simulink model "MCLV_Board_33Fj256MC710A_BLDC_wHall_async_2_10Khz"  (Simulink 7.5)
settings: Solver=FixedStepDiscrete  StartTime=0.0  StopTime=10.0  FixedStep=.001  RelTol=1e-3
undefined symbols (not defined in the file or in its folder): CN19max, D13, D14, D15, DiscIntNeverNeededParam, F13, Max, ms, Pin, PWM1max, PWMmax, Resol, us
libraries: MCHP_Blockset x17, simulink x8
CloseFcn:
  | rtwprivate ssgencode ModelCloseRequest MCLV_Board_33Fj256MC710A_BLDC_wHall_async_2_10Khz
settings Model: Creator=Lubin Kerhuel  LastModifiedBy=Lubin Kerhuel
settings OptimizationCC: InlineParams=on  InlineInvariantSignals=on  EnhancedBackFolding=on  OptimizeModelRefInitCode=on  LifeSpan=1
settings HardwareCC: ProdBitPerInt=16  ProdIntDivRoundTo=Zero  ProdEndianess=LittleEndian  ProdWordSize=16  ProdHWDeviceType=Generic->Custom
settings ModelReferenceCC: ModelReferenceNumInstancesAllowed=Single
settings RTWCC: SystemTargetFile=MCHP_dsPIC_stf.tlc  TemplateMakefile=MCHP_dsPIC.tmf  Description=Microchip Embedded Target PIC24 dsPIC30 dsPIC33 (real-time)  GenerateReport=on  ProcessScript=MCHP_dsPIC_stf_make_rtw_hook  IncludeHyperlinkInReport=on  GenerateTraceInfo=on  GenerateTraceReport=on  GenerateTraceReportSl=on  GenerateTraceReportSf=on  GenerateTraceReportEml=on
settings CodeAppCC: IgnoreCustomStorageClasses=off  MaxIdLength=255
settings STFCustomTargetCC: TargetLibSuffix=_lib.a  IncludeMdlTerminateFcn=off  CombineOutputUpdateFcns=on  SuppressErrorStatus=on  ERTCustomFileBanners=on  SupportContinuousTime=off  SystemTargetFile=MCHP_dsPIC_stf.tlc
settings ERTTargetCC: TargetLibSuffix=_lib.a  MultiwordLength=2048  ParMdlRefBuildCompliant=off  CompOptLevelCompliant=off  IncludeMdlTerminateFcn=off  SuppressErrorStatus=on  ERTFirstTimeCompliant=off  SupportNonInlinedSFcns=on  ModelStepFunctionPrototypeControlCompliant=off  CPPClassGenCompliant=off  InlinedParameterPlacement=NonHierarchical  ERTSrcFileBannerTemplate=MCHP_dsPIC_code_template.cgt  ERTHdrFileBannerTemplate=MCHP_dsPIC_code_template.cgt  ERTDataSrcFileTemplate=MCHP_dsPIC_code_template.cgt  ERTDataHdrFileTemplate=MCHP_dsPIC_code_template.cgt  ERTCustomFileTemplate=MCHP_main.tlc  ConvertIfToSwitch=off
settings CustomProperty: DataType=string  Value=33FJ256MC710A
settings EnumStrPairs: String=elf

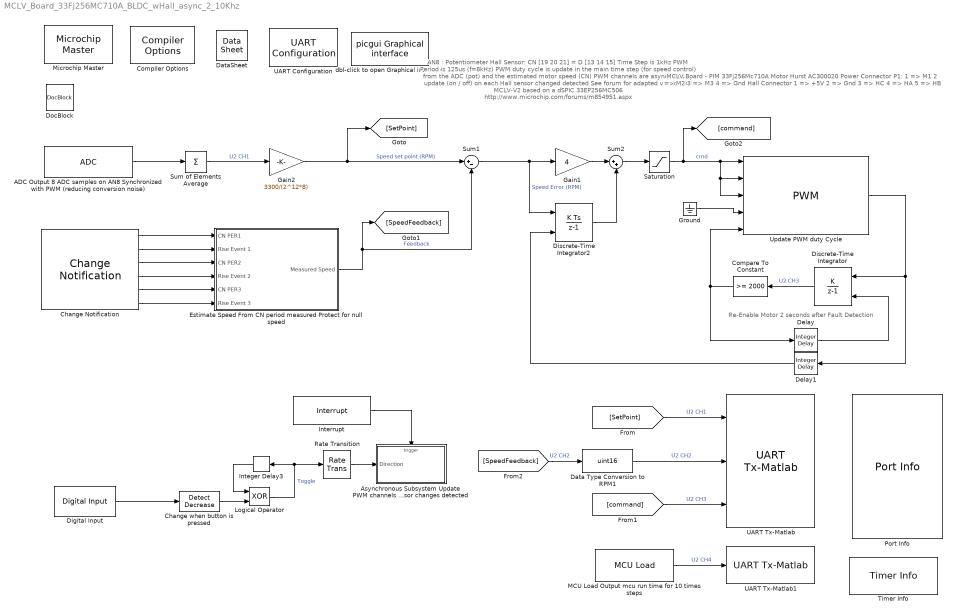
== system MCLV_Board_33Fj256MC710A_BLDC_wHall_async_2_10Khz ==
  note: Re-Enable Motor 2 seconds after Fault Detection
  note: AN8 : Potentiometer
      | Hall Sensor: CN [19 20 21] = D [13 14 15]
      |
      | Time Step is 1kHz
      | PWM Period is 125us (f=8kHz)
      | PWM duty cycle is update in the main time step (for speed control)
      | from the ADC (pot) and the estimated motor speed (CN)
      | PWM channels are asynchrousnly update (on / off) on each Hall sensor changed detected
      |
      | See forum for adapted version for MCLV-V2 based on a dSPIC 33EP256MC506
      | http://www.microchip.com/forums/m854951.aspx
  note: MCLV Board -  PIM 33Fj256Mc710A
      | Motor Hurst AC300020
      | Power Connector P1:
      | 1 => M1
      | 2 => M2
      | 3 => M3
      | 4 => Gnd
      | Hall Connector
      | 1 => +5V
      | 2 => Gnd
      | 3 => HC
      | 4 => HA
      | 5 => HB
  ADC Output 8 ADC samples on AN8 Synchronized with PWM (reducing conversion noise) : MCHP_Blockset/Analog IO/ADC  ADC_REF=1  Mode=12 bits  FORM=0000 dddd dddd dddd ==> Unsigned integer  nSAMPLECHANNELS=CH0 only  nSAMPLECHANNELS_12bits=CH0 only  SIMULTANEOUS=in Sequence  ADxCSS=8  MUXA_CH0N=off  MUXA_CH123=Dynamic Options  MUXA_CH123_TXT=AN0 : AN1 : AN2  MUXB_CH0=AN1  MUXB_CH0N=on  MUXB_CH123=Dynamic Options  MUXB_CH123_TXT=AN0 : AN1 : AN2  SequenceRepeat=8  SequenceTiming=are done as fast as possible ; triggered by user define source  SSRC_SSRCG=Dynamic Options  SSRC_SSRCG_TXT=6  Update_BlockOutput=After all trig and conversion sequence  Trig_TimeStep=with each update of the ADC block output  ADC_DMA_CHANNEL=use DMA Channel 1  SampleTime=0.001  Info=Total Time for Sample & Conversion : 7.56e-005s including 0s (x 8) sample time.  MCHP_PORT={Analog Input 8}{AN8}15:2:B8;  MCHP_MASTERLINK=MCLV_Board_33Fj256MC710A_BLDC_wHall_async_2_10Khz/Microchip Master  ADC_TIMING=[7.5599999999999994e-005]
  Asynchronous Subsystem Update PWM channels to On / Off based on Hall sensor changes detected : Subsystem
  Change Notification : MCHP_Blockset/Pulse Input//Output/Change Notification  IntPriority=6  Channel="[19    20    21]"  Channel_EP="[  D13  D14  D15 ]"  Channel_OLD="[19  20  21]"  Channel_UP_Down_Periode="[4     4     4]"  MaxChannel="[0.25   0.25   0.25]"  SafeMarge="[200   200   200]"  MaxChannelValue="2.^[ 15.253  15.253  15.253]  =>  [39062  39062  39062]"  CNxmax="[39062  39062  39062]"  Timer="[2  2  2]"  ChangeDetected="[1     1     1]"  OutputPortValue="[0     0     0]"  SampleTime=.001  Status=OK  MCHP_PORT={Change Notification 19}{CN19}9:0:D13;{Change Notification 20}{CN20}9:0:D14;{Change Notification 21}{CN21}9:0:D15;  MCHP_TIMER_REQUEST={Change Notification 19}{CN19}7:1:1:0:[]:30000000;{Change Notification 20}{CN20}7:1:1:0:[]:30000000;{Change Notification 21}{CN21}7:1:1:0:[]:30000000;  MCHP_TIMER_RESULT=[2 117186.50000000007 ;2 117186.50000000007 ;2 117186.50000000007 ]  MCHP_USER_INTERRUPTS={CNIE}{CN}{Change Notification}{6};  MCHP_MASTERLINK=MCLV_Board_33Fj256MC710A_BLDC_wHall_async_2_10Khz/Microchip Master
  Change when button is pressed : simulink/Logic and Bit Operations/Detect Decrease  SystemSampleTime=-1  vinit=0.0
  Compare To Constant : simulink/Logic and Bit Operations/Compare To Constant  SystemSampleTime=-1  relop=>=  const=2000  LogicOutDataTypeMode=boolean
  Compiler Options : MCHP_Blockset/System Configuration/Compiler Options  Priority=1  LATEST_CMPLR=on  COMP_LIST=Dynamic Options  COMP_LIST_TXT=xc16 - v1.26  USE_64BIT_DOUBLE=off  MCHP_MULTITHREAD_COMPILATION=on  MCHP_MASTERLINK=MCLV_Board_33Fj256MC710A_BLDC_wHall_async_2_10Khz/Microchip Master  OPTIMIZATION_LEVEL=3  MPLAB_LINKLIB=default  MPLAB_LINKLIB1=default  UNROLL_LOOPS=off  OMIT_FRAME_POINTER=off  PROCEDURAL_ABSTRACTION=off  MCONST=in data memory  MDATA=Use only memory below address 8192 (faster)  MSCALAR=Use only memory below address 8192 (faster)  MCODE=is less than 32768 (faster)  HEAP_SIZE=0  OMF=elf  DEBUG_INFO=on  AssemblyListing=off  ProduceHexOutput=on
  Data Type Conversion to RPM1 : DataTypeConversion  OutDataTypeMode=uint16  OutDataTypeStr=uint16  SaturateOnIntegerOverflow=on
  DataSheet : MCHP_Blockset/System Info/Data Sheet  DOC_Type=datasheet  DOC_MCHP_Id=33FJ256MC710A  DOC_FilePath=C:\Users\Lubin Kerhuel\AppData\Local\Temp\70594d.pdf  DOC_FileLastCheckTime="[2012              9              2             21             45         49.233]"  cpy_MCHP_Id=33FJ256MC710A  MCHP_MASTERLINK=MCLV_Board_33Fj256MC710A_BLDC_wHall_async_2_10Khz/Microchip Master
      settings: AttributesFormatString=%<cpy_MCHP_Id>
  Delay : simulink/Discrete/Integer Delay  vinit=0  samptime=-1  NumDelays=1
  Delay1 : simulink/Discrete/Integer Delay  vinit=0  samptime=-1  NumDelays=1
  Digital Input : MCHP_Blockset/Digital IO/Digital Input  PORT=Dynamic Options  PORT_TXT="D   [ 0 : 15 ]"  PIN=6  PACK=off  SIMULTANEOUS=off  ORDERING=None  SampleTime=.01  MCHP_PORT={Digital In}{DIN}2:0:D6;  MCHP_MASTERLINK=MCLV_Board_33Fj256MC710A_BLDC_wHall_async_2_10Khz/Microchip Master
  Discrete-Time Integrator : DiscreteIntegrator  IntegratorMethod=Accumulation: Forward Euler  gainval=1  ExternalReset=level  SampleTime=-1  OutDataTypeMode=uint16  OutDataTypeStr=uint16  SaturateOnIntegerOverflow=on  UpperSaturationLimit=0  LowerSaturationLimit=0  ICPrevOutput=DiscIntNeverNeededParam  ICPrevScaledInput=DiscIntNeverNeededParam
  Discrete-Time Integrator2 : DiscreteIntegrator  gainval=16  ExternalReset=level  SampleTime=-1  OutMin=[-PWMmax]  OutMax=[PWMmax]  OutDataTypeMode=Specify via dialog  OutDataType=fixdt(1,16,1)  OutDataTypeStr=fixdt(1,16,1)  SaturateOnIntegerOverflow=on  LimitOutput=on  UpperSaturationLimit=PWM1max  LowerSaturationLimit=0  ICPrevOutput=DiscIntNeverNeededParam  ICPrevScaledInput=DiscIntNeverNeededParam
  DocBlock : simulink/Model-Wide Utilities/DocBlock  SystemSampleTime=-1  DocumentType=Text
  Estimate Speed From CN period measured Protect for null speed : Subsystem
  Gain1 : Gain  Gain=4  ParameterDataTypeMode=Specify via dialog  ParameterDataType=fixdt(1,16,10)  ParamDataTypeStr=fixdt(1,16,10)  OutDataTypeMode=int16  OutDataTypeStr=int16  RndMeth=Round  SaturateOnIntegerOverflow=on
  Gain2 : Gain  Gain=3300/(2^12*8)  ParamDataTypeStr=Inherit: Inherit from 'Gain'  OutDataTypeMode=uint16  OutDataTypeStr=uint16  RndMeth=Round  SaturateOnIntegerOverflow=on
  Ground : Ground
  Integer Delay3 : simulink/Discrete/Integer Delay  vinit=1  samptime=-1  NumDelays=1
  Interrupt : MCHP_Blockset/System Functions/Interrupt  IntPriority=6  Interruption=Dynamic Options  Interruption_TXT=Change Notification  Status=OK  StartupExecute=off  MCHP_MASTERLINK=MCLV_Board_33Fj256MC710A_BLDC_wHall_async_2_10Khz/Microchip Master
  Logical Operator : Logic  Operator=XOR  AllPortsSameDT=off  OutDataTypeMode=boolean  OutDataTypeStr=boolean
  MCU Load Output mcu run time for 10 times steps : MCHP_Blockset/Profiling/MCU Load  MCULoadPin=Dynamic Options  MCULoadPin_TXT=F13 / Pin[39]  MCULoadMeasure=on  TIMER_Resolution=Dynamic Options  TIMER_Resolution_TXT="Resol: 0.2(us)  -  Max: 13.1(ms)"  MCHP_PORT={MCU Load Pin}{MCU_Load}0:1:F13;  MCHP_TIMER_REQUEST={MCU_Load}{MCU_Load}21:5:0:0:[]:524288;  MCHP_TIMER_RESULT=[1 65535 ]  MCHP_MASTERLINK=MCLV_Board_33Fj256MC710A_BLDC_wHall_async_2_10Khz/Microchip Master  MCHP_COMPILED_INFO="CompiledSampleTime= [0.01   0 ];CompiledInportDataTypes=[ ];CompiledInportDataWidth=[];"  Info="Timer 1:  Resol: 200(ns)  -  Max: 13.1072(ms)"  SampleTime=.01
  Microchip Master : MCHP_Blockset/System Configuration/Microchip Master  PICREF=33FJ256MC710A  TIMESTEP_REF=ADC  BUSYFLAG=Dynamic Options  BUSYFLAG_TXT=None  PWRTEN=PWRT enabled  BOREN=Disable  BODENV=2.7V  BORV=Brown-out Reset set at 2.0V  FPWRT=128ms  DSBOREN=Deep Sleep BOR enabled in Deep Sleep  DSLPBOR=Deep Sleep BOR enabled in Deep Sleep  MCLRE=Enabled  SMCLR=MCLR pin generates a normal system Reset  PMDL1WAY=Allow only one reconfiguration  RSTPRI=Device will obtain reset instruction from Primary flash  TEMP=Not used  SOSCSRC=Analog Mode for use with crystal  SOSCSEL=Secondary oscillator configured for high-power operation  IOL1WAY=Allow only one reconfiguration  ALTVREF=Voltage reference input; ADC =RA9/RA10 Comparator =RA9;RA10  DISUVREG=Regulator is disabled  DSSWEN=Deep Sleep is controlled by the register bit DSEN  LPCFG=Disabled - regardless of RETEN  RTCBAT=RTC operation is continued through VBAT  VBTBOR=VBAT BOR enabled  WUTSEL=Default regulator start-up time used  POWERSAVE=off  FNOSC=Primary oscillator (XT; HS; EC)  FPR=ECIO w/ PLL 16x  FOSFPR=HS3 w/PLL 16x  FOS=Primary Oscillator  FRANGE=High Range  OSCILLATOR_SELECT=Crystal / Ceramic resonator  OSCILLATOR_SELECT_spd=Crystal / Ceramic resonator  QUARTZ=8e6  QUARTZ_spd=8e6  POSCGAIN=2x gain setting  POSCBOOST=Boost the kick start of the oscillator  SOSCGAIN=2x gain setting  SOSCBOOST=Boost the kick start of the oscillator  ACTIV_PLL=on  ACTIV_PLL_spd=on  MIPS_DESIRED=40e6  MIPS_DESIRED_spd=40e6  FPLLMUL=24x Multiplier  FPLLIDIV=12x Divider  POSCFREQ=Primary oscillator/external clock input frequency greater than 8MHz  POSCMD=XT Oscillator Mode  POSCMOD=Primary Oscillator Disabled  MIPS=40 * 1e6  FPLLODIV=PLL Divide by 256  PLLKEN=Clock switch to PLL source will wait until the PLL lock signal is valid.  FCKSM=Clock switching is enabled; Fail-Safe Clock Monitor is disabled  FCKSMEN=Sw Disabled; Mon Disabled  IESO=Start up with FRC; then switch  DSWDTPS=1:2;147;483;648 (25.7 Days)  FWDTEN=Disable  FWDTWINSZ=Window size is 25%  FWPSA=1:512  FWPSA0=1:128  FWPSB=1:16  WDT=Disable  WDTPOST=1:32768  WDTPRE=1:128  WDTPS=1:32768  WINDIS=Watchdog Timer in Non-Window mode  WWDTEN=Non-Window mode  DSWDTEN=DSWDT enabled  DSWDTOSC=DSWDT uses Low Power RC Oscillator (LPRC)  FPBDIV=Pb_Clk is Sys_Clk/8  FSOSCEN=Enabled  LPRCSEL=High Power; High Accuracy Mode  OSCIOFCN=OSCO/CLKO/RA3 functions as CLKO (FOSC/2)  OSCIOFNC=OSC2 pin has digital I/O function  LVRCFG=Low Voltage regulator is not available  PLL_96MHZ=Enabled  PLL96MHZ=96 MHz PLL Startup is enabled automatically on start-up  PLLDIV=PLL is disabled  WDTCLK=WDT uses LPRC  WDTCMX=WDT clock source is determined by the WDTCLK Configuration bits  WDTWIN=WDT Window is 25% of WDT period  APL=Aux Flash Code protect is disabled  APLK=Aux Flash Write Protection or Code Protection is Enabled  AWRP=Aux Flash may be written  BSS=No boot program Flash segment  BWP=Protection Disabled  BWRP=Boot Segment may be written  CP=Protection Disabled  EBS=No Boot EEPROM  ESS=No Segment Data EEPROM  GCP=General Segment Code protect is disabled  GSS=User program memory is not code-protected  GSS0=No protection  GSSK=General Segment Write Protection or Code Protection is Enabled  GWRP=General Segment may be written  PWP=Disable  RBS=No Boot RAM  RSS=No Secure RAM  SSS=No Secure Segment  SWRP=Secure segment may be written  WPCFG=Disable  WPDIS=Disable  WPEND=Write Protect from WPFP to the last page of memory  WPFP=Page 127 (0x1FC00)  ICESEL=Communicate on PGEC1/PGED1  ICS=Communicate on PGEC1 and PGED1  JTAGEN=Disable  COE=Reset Into Operational Mode  RES=Not used  DEBUG=Debugger is disabled  BACKBUG=Not used  BKBUG=Device resets into Operational mode  ALTI2C=I2C mapped to SDA1/SCL1 pins  ALTI2C1=I2C1 mapped to SDA1/SCL1 pins  ALTI2C2=I2C2 mapped to SDA2/SCL2 pins  ALTQIO=QEA1; QEB1; INDX1 are selected as inputs to QEI1  ALTSS1=SS1A is selected as the I/O pin for SPI1  CMPPOL0=Hysteresis is applied to falling edge  CMPPOL1=Hysteresis is applied to falling edge  FCANIO=Default CAN I/O  FETHIO=Default Ethernet I/O  FMIIEN=MII Enabled  FSRSSEL=SRS Priority 7  FUSBIDIO=Controlled by the USB Module  FVBUSONIO=Controlled by USB Module  HPOL=PWM module high side output pins have active-high output polarity  HYST0=45 mV Hysteresis  HYST1=45 mV Hysteresis  I2C1SEL=Use Default SCL1/SDA1 Pins For I2C1  LPOL=Active High  PWMPIN=PWM module pins controlled by PWM module at device Reset  RTCOSC=RTCC uses Secondary Oscillator (SOSC)  UPLLEN=Disabled and bypassed  UPLLIDIV=12x Divider  ATMOD8=Not used  ALTPMP=EPMP pins are in default location mode  I2C2SEL=I2C2 is multiplexed to SDA2/RA3 and SCL2/RA2  ALTADREF=AVREF+/AVREF- are mapped to RA9/RA10  ALTCVREF=CVREF+/CVREF- are mapped to RA9/RA10  PWMLOCK=PWM registers may be written without key sequence  MCHP_TIMER_RESULT=[ ]  MCHP_PLLRegisters="[5    138  16385     -1]"  MCHPVAR=MCHP.fcy.periph=40000000;MCHP.fcy.MIPS=40000000;MCHP.PowerSave=0;MCHP.TimeStepFactor=-1000;MCHP.TimeStep_Timer=-1;MCHP.NTIMERS=9;MCHP.id.name='33FJ256MC710A';MCHP.id.N=reshape([33 256 710],1,3);MCHP.id.L=reshape({ 'FJ','MC','A'},1,3);MCHP.id.Arch=3;MCHP.periph.PPS.reg_RPINRx=reshape(MCHP_Fun.Hex2num('[]'),0,0);MCHP.PPS.dsPIC.RP=reshape(MCHP_Fun.Hex2num('[]'),0,0);MCHP.PPS.dsPIC.RPI=reshape(MCHP_Fun.Hex2num('[]'),0,0);MCHP.PPS.dsPIC.RPINR_list=reshape({ '1','INT1','INT2','INT3','INT4','T1CK','T2CK','T3CK','T4CK','T5CK','T6CK','T7CK','T8CK','T9CK','IC1','IC2','IC3','IC4','IC5','IC6','IC7','IC8','OCFA','OCFB','FLT1','FLT2','FLT3','FLT4','QEA1','QEB1','INDX1','HOME1','QEA2','QEB2','INDX2','HOME2','U1RX','U1CTS','U2RX','U2CTS','SDI1','SCK1','SS1','44','SDI2','SCK2','SS2','48','CSDIR','CSCK','COFS','52','C1RX','C2RX','U3RX','U3CTS','U4RX','U4CTS','SDI3','SCK3','SS3','62','SDI4','SCK4','SS4','66','IC9','IC10','IC11','IC12','IC13','IC14','IC15','IC16','OCFC','SYNCI1','SYNCI2','DTCMP1','DTCMP2','DTCMP3','DTCMP4','DTCMP5','DTCMP6','DTCMP7','FLT5','FLT6','FLT7','FLT8','89','SENT1','SENT2','92'},1,92);MCHP.PPS.dsPIC.RPOR_list=reshape({ '1','C1OUT','C2OUT','U1TX','U1RTS','U2TX','U2RTS','SDO1','SCK1','SS1','SDO2','SCK2','SS2','CSDO','CSCK','COFS','C1TX','17','OC1','OC2','OC3','OC4','22','23','24','25','UPDN1','UPDN2'},1,28);MCHP.PPS.map_RPnR_RPORx=reshape(MCHP_Fun.Hex2num('[]'),0,0);MCHP.Rx=reshape([17 25 -1 72 93 87 90 -1 -1 -1 -1 38 24 6 76 94 88 89 -1 -1 -1 -1 58 23 7 77 98 52 57 -1 -1 -1 -1 59 22 8 78 99 51 56 -1 -1 -1 -1 60 21 9 81 100 49 -1 -1 -1 -1 -1 61 20 -1 82 3 50 -1 -1 -1 -1 -1 91 26 -1 83 4 55 10 -1 -1 -1 -1 92 27 -1 84 5 54 11 -1 -1 -1 -1 -1 32 -1 68 18 53 12 -1 -1 -1 -1 28 33 -1 69 19 -1 14 -1 -1 -1 -1 29 34 -1 70 -1 -1 -1 -1 -1 -1 -1 -1 35 -1 71 -1 -1 -1 -1 -1 -1 -1 -1 41 63 79 -1 40 96 -1 -1 -1 -1 -1 42 73 80 -1 39 97 -1 -1 -1 -1 66 43 74 47 -1 -1 95 -1 -1 -1 -1 67 44 64 48 -1 -1 1 -1 -1 -1 -1],11,16);MCHP.ADC.ANtype=reshape([3 1],1,2);MCHP.ADC.ADCONx=reshape([47087 59327 40959 7 0 0],1,6);MCHP.ADC.ADCHS_0=reshape([40863 1799],1,2);MCHP.ADC.Flags=reshape([1 0],1,2);MCHP.ADC.Buffer=reshape([1 1],1,2);MCHP.ADC.port=reshape([16 17 18 19 20 21 22 23 24 25 26 27 28 29 30 31 33 34 35 36 72 73 6 7 -1 -1 -1 -1 -1 -1 -1 -1 -1 -1 -1 -1 -1 -1 -1 -1 -1 -1 -1 -1 -1 -1 -1 -1 -1 -1 -1 -1 -1 -1 -1 -1 -1],1,57);MCHP.ADC.port_VrefP=-1;MCHP.ADC.port_VrefM=-1;MCHP.ADC.port_AVdd=-1;MCHP.ADC.port_AVss=-1;MCHP.memory.RAM=30720;MCHP.memory.RAM_XBegin=2048;MCHP.memory.RAM_YBegin=18432;MCHP.memory.RAM_dma=reshape([30720 32768],1,2);MCHP.DMA.Num=8;MCHP.DMA.CNTmax=65535;MCHP.QEI.QEICONx=reshape([49151 -1 -1 -1 -1 -1],1,6);MCHP.QEI.QEItype=0;MCHP.QEI.Port_QEI_INDX=reshape([19 -1],1,2);MCHP.QEI.Port_QEI_QEA=reshape([20 -1],1,2);MCHP.QEI.Port_QEI_QEB=reshape([21 -1],1,2);MCHP.QEI.Port_QEI_UPDN=reshape([55 -1],1,2);MCHP.INT.Port=reshape([86 72 73 14 15],1,5);MCHP.PWM_HS.Flags=reshape([0 0 0],1,3);MCHP.PWM.port_FLT=reshape([72 73 -1 -1 -1 -1 -1 -1 -1 -1 -1 -1 -1 -1 -1 -1 -1 -1 -1 -1 -1 -1 -1 -1 -1 -1 -1 -1 -1 -1 -1 -1 -1],1,33);MCHP.PWM.PWMRef=1;MCHP.PWM.Flag=7;MCHP.PWM.Port_PWM_l=reshape([64 -1 66 -1 68 -1 70 -1 -1 -1 -1 -1 -1 -1 -1 -1 -1 -1],2,9);MCHP.PWM.Port_PWM_h=reshape([65 -1 67 -1 69 -1 71 -1 -1 -1 -1 -1 -1 -1 -1 -1 -1 -1],2,9);MCHP.IC.Port=reshape([56 57 58 59 60 61 62 63 0 0 0 0 0 0 0 0],1,16);MCHP.IC.type=0;MCHP.OC.Port=reshape([48 49 50 51 52 53 54 55 0 0 0 0 0 0 0 0],1,16);MCHP.OC.type=0;MCHP.CN.Port=reshape([46 45 16 17 18 19 20 21 102 103 104 105 31 52 53 54 55 84 85 61 62 63 6 7 -1 -1 -1 -1 -1 -1 -1 -1 -1 -1 -1 -1 -1 -1 -1 -1 -1 -1 -1 -1 -1 -1 -1 -1 -1 -1 -1 -1 -1 -1 -1 -1 -1 -1 -1 -1 -1 -1 -1 -1 -1 -1 -1 -1 -1 -1 -1 -1 -1 -1 -1 -1 -1 -1 -1 -1 -1 -1 -1 -1 -1],1,85);MCHP.CN.PullUp=reshape([65535 255 0 0 0 0 0 0 0 0 0],1,11);MCHP.CN.type=0;MCHP.CN.Flag_PullDown=1;MCHP.SPI.Refs=reshape([1 2 0 0 0 0],1,6);MCHP.SPI.SPIxCON1=8191;MCHP.SPI.SPIxCON2=57346;MCHP.SPI.Port_SDI=reshape([87 103 -1 -1 -1 -1],1,6);MCHP.SPI.Port_SDO=reshape([88 104 -1 -1 -1 -1],1,6);MCHP.SPI.Port_SCK=reshape([86 102 -1 -1 -1 -1],1,6);MCHP.SPI.Port_SS=reshape([18 105 -1 -1 -1 -1],1,6);MCHP.I2C.Refs=reshape([1 2 0 0 0],1,5);MCHP.I2C.I2CxCON=49151;MCHP.I2C.NewRegName=1;MCHP.I2C.Port_SDA=reshape([99 3 -1 -1 -1],1,5);MCHP.I2C.Port_SCL=reshape([98 2 -1 -1 -1],1,5);MCHP.I2C.Port_ASDA=reshape([-1 -1 -1 -1 -1],1,5);MCHP.I2C.Port_ASCL=reshape([-1 -1 -1 -1 -1],1,5);MCHP.I2C.Fuse_Port_SCL_SDA=reshape([-1 -1 -1 -1 -1 -1 -1 -1 -1 -1],2,5);MCHP.I2C.Fuse_Port_ASCL_ASDA=reshape([-1 -1 -1 -1 -1 -1 -1 -1 -1 -1],2,5);MCHP.Comp.Port_CVrefin=-1;MCHP.Comp.Port_CVref=-1;MCHP.Comp.Port_CVref1O=-1;MCHP.Comp.Port_CVref2O=-1;MCHP.Comp.Port_CxOUT=reshape([-1 -1 -1 -1 -1],1,5);MCHP.Comp.Port_OAxOUT=reshape([-1 -1 -1 -1 -1],1,5);MCHP.Comp.Port_CxINP=reshape([-1 -1 -1 -1 -1],1,5);MCHP.Comp.Port_CxINM=reshape([-1 -1 -1 -1 -1 -1 -1 -1 -1 -1 -1 -1 -1 -1 -1 -1 -1 -1 -1 -1],4,5);MCHP.Comp.nComp=reshape([0 0 0],1,3);MCHP.Comp.OpAmp=0;MCHP.Comp.CVRCON=reshape([0 0],1,2);MCHP.UART.port_Rx=reshape([82 84 -1 -1 -1 -1],1,6);MCHP.UART.port_Tx=reshape([83 85 -1 -1 -1 -1],1,6);MCHP.UART.port_ARx=reshape([-1 -1],1,2);MCHP.UART.port_ATx=reshape([-1 -1],1,2);MCHP.UART.port_RTS=reshape([63 93 -1 -1 -1 -1],1,6);MCHP.UART.port_CTS=reshape([62 92 -1 -1 -1 -1],1,6);MCHP.UART.reg_UxMODE=reshape([48127 48127 -1 -1 -1 -1],1,6);MCHP.UART.reg_UxSTA=reshape([61439 61439 -1 -1 -1 -1],1,6);  MCHP_CRC=4181521  BTMODE=Device is in Single Boot (legacy) mode  RES1=Not used  PLLSS=PLL is fed by the Primary oscillator  RES2=Not used  ALTCMPI=C1INC is on RB13; C2INC is on RB9 and C3INC is on RA0  BOREN1=BOR Enabled [When BOREN=1]  ALTRB6=Append the RP6/ASCL1/PMPD6 functions of RB6 to RA1 pin functions  RETCFG=Retention regulator is not available  DFMCY=Not used  BSS2=No Boot Segment  BSEN=No Boot Segment  CWRP=Configuration Segment may be written  CSS=No Protection (other than CWRP)  AIVTDIS=Disable Alternate Vector Table  BSLIM=Not used  WDTEN=Disable  BTSWP=Not used  DBCC=Not used  CTXT1=Not Assigned  CTXT2=Not Assigned  SEQNUM=Not used  nSEQNUM=Not used  BOREN0=Enabled  DMTIVT=Not used  DMTCNT=2^31 (2147483648)  DMTEN=Dead Man Timer is Enabled and cannot be disabled by software  ON=Not used  USERID=Not used  RESERVED1=Not used  PGL1WAY=Allow only one reconfiguration  FPLLRNG=34-68 MHz Input  FPLLICLK=FRC is input to the System PLL  FPLLMULT=PLL Multiply by 128  UPLLFSEL=USB PLL input is 24 MHz  DMTINTV=Window/Interval value is 127/128 counter value  WDTSPGM=WDT stops during Flash programming  FDMTEN=Deadman Timer is disabled  TRCEN=Trace features in the CPU are enabled  BOOTISA=Boot code and Exception code is MIPS32  FECCCON=ECC and Dynamic ECC are disabled (ECCCON bits are writable)  EXTDDRSIZE=External DDR2 Size is 128 MB  FSLEEP=Flash is powered down when the device is in Sleep mode  DBGPER=Allow CPU access to all permission regions  EJTAGBEN=Normal EJTAG functionality  TSEQ=Not used  CSEQ=Not used
  Port Info : MCHP_Blockset/System Info/Port Info  MCHP_MASTERLINK=MCLV_Board_33Fj256MC710A_BLDC_wHall_async_2_10Khz/Microchip Master
  Rate Transition : RateTransition  Integrity=off  Deterministic=off
  Saturation : Saturate  UpperLimit=PWM1max  LowerLimit=0  OutDataTypeMode=uint16  OutDataTypeStr=uint16
  Sum of Elements Average : Sum  Inputs=+  AccumDataTypeStr=uint16  OutDataTypeMode=uint16  OutDataTypeStr=uint16
  Sum1 : Sum  Inputs=|+-  AccumDataTypeStr=fixdt(1,16,2)  OutDataTypeMode=Specify via dialog  OutDataType=fixdt(1,16,2)  OutDataTypeStr=fixdt(1,16,2)  SaturateOnIntegerOverflow=on
  Sum2 : Sum  Inputs=|++  AccumDataTypeStr=int16  OutDataTypeMode=uint16  OutDataTypeStr=uint16  SaturateOnIntegerOverflow=on
  Timer Info : MCHP_Blockset/System Info/Timer Info  MCHP_MASTERLINK=MCLV_Board_33Fj256MC710A_BLDC_wHall_async_2_10Khz/Microchip Master
  UART Configuration : MCHP_Blockset/BUS UART/UART Configuration  UART_REF=2  BAUD_Choice=Dynamic Options  BAUD_Choice_TXT="115200         [-0.22%]"  BAUD_Choice_IR=Dynamic Options  BAUD_Choice_IR_TXT=[]  BAUD_Custom=115200  IRDA=off  ALT_IO=on  PIN_RX=Dynamic Options  PIN_RX_TXT=Dynamic Options  PIN_TX=Dynamic Options  PIN_TX_TXT=Dynamic Options  FlowControl=None  PIN_CTS=Dynamic Options  PIN_CTS_TXT=Dynamic Options  PIN_RTS=Dynamic Options  PIN_RTS_TXT=Dynamic Options  MCHP_PORT="{UART2  Rx}{U2RX}3:0:F4;{UART2  Tx}{U2TX}3:1:F5;"  MCHP_MASTERLINK=MCLV_Board_33Fj256MC710A_BLDC_wHall_async_2_10Khz/Microchip Master  MCHP_COM_ExtPil=off  TX_IMPLEMENTATION=Circular Buffer  TX_INT_PRIORITY=5  TX_INT_WHEN=is empty  TX_CIRCULAR_SIZE=32  TX_DMA_CHANNEL="0   (Lowest Priority)"  TX_DMA_SIZE=32  RX_IMPLEMENTATION=Circular Buffer  RX_INT_PRIORITY=1  RX_INT_WHEN=receive 1 character  RX_CIRCULAR_SIZE=32  InitSequence_chkbox=off  BAUD_Choice_InitSeq=Dynamic Options  BAUD_Choice_InitSeq_TXT="110         [+0.00%]"  BAUD_Choice_IR_InitSeq=Dynamic Options  BAUD_Choice_IR_InitSeq_TXT=0  BAUD_Custom_InitSeq=0  InitSequence='Hello World'
  UART Tx-Matlab : MCHP_Blockset/BUS UART/UART Tx-Matlab  UART_REF=2  CHANNELS="[1  2 3]"  AllOrNothing=off  SampleTime=-1  MCHP_MASTERLINK=MCLV_Board_33Fj256MC710A_BLDC_wHall_async_2_10Khz/Microchip Master  MCHP_COMPILED_INFO="CompiledSampleTime= [0.001   0 ];CompiledInportDataTypes=[  5   5   5 ];CompiledInportDataWidth=[1  1  1];"
  UART Tx-Matlab1 : MCHP_Blockset/BUS UART/UART Tx-Matlab  UART_REF=2  CHANNELS=4  AllOrNothing=off  SampleTime=-1  MCHP_MASTERLINK=MCLV_Board_33Fj256MC710A_BLDC_wHall_async_2_10Khz/Microchip Master  MCHP_COMPILED_INFO="CompiledSampleTime= [0.01   0 ];CompiledInportDataTypes=[  5 ];CompiledInportDataWidth=[1];"
  Update PWM duty Cycle : MCHP_Blockset/PWM IO/PWM  PWM_REF=1  ChannelHighLowChk=off  Channel="[1  2 3]"  ChannelHigh=[1 2 4]  InitialPeriod=.001/8  InputPeriodeChk=off  CAM=off  IUE=off  Info="PWM1max = 9997  ;   % ==>  13.2873 bits"  MCHP_MASTERLINK=MCLV_Board_33Fj256MC710A_BLDC_wHall_async_2_10Khz/Microchip Master  MCHP_PORT={PWM Fault A}{FLTA}5:0:E8;{PWM_L1}{PWM_L}5:1:E0;{PWM_L2}{PWM_L}5:1:E2;{PWM_L3}{PWM_L}5:1:E4;{PWM_H1}{PWM_H}5:1:E1;{PWM_H2}{PWM_H}5:1:E3;{PWM_H3}{PWM_H}5:1:E5;  ADC_VARTRIG={PWM Primary Special Event Trigger;6}  SampleTime=-1  DeadTimePrescaleA=2e-6  DeadTimePrescaleB=0  DTPWM1a=Prescaler A  DTPWM1i=Prescaler A  DTPWM2a=Prescaler A  DTPWM2i=Prescaler A  DTPWM3a=Prescaler A  DTPWM3i=Prescaler A  DTPWM4a=Prescaler A  DTPWM4i=Prescaler A  PIN_FaultA=Dynamic Options  PIN_FaultA_TXT=<empty>  FAULTA_FLATM=Use Re-Enable block input after Fault is detected  FaultA_Output=on  FaultA_PWM1_State=H/L ==> 00  FaultA_PWM2_State=H/L ==> 00  FaultA_PWM3_State=H/L ==> 00  FaultA_PWM4_State=No Changes (PWM)  PIN_FaultB=Dynamic Options  PIN_FaultB_TXT=<empty>  FAULTB_FLBTM=Use Re-Enable block input after Fault is detected  FaultB_Output=off  FaultB_PWM1_State=No Changes (PWM)  FaultB_PWM2_State=No Changes (PWM)  FaultB_PWM3_State=No Changes (PWM)  FaultB_PWM4_State=No Changes (PWM)  PxSECMP=0  PxSECMPBlkInChk=off  OVDCONChk=on
  dbl-click to open Graphical interface : MCHP_Blockset/BUS UART/picgui Graphical interface  Nothing=0
  wires:
  Update PWM duty Cycle/1 -> Discrete-Time Integrator/1, Delay1/1
  Discrete-Time Integrator/1 -> Compare To Constant/1  "U2 CH3"
  Compare To Constant/1 -> Update PWM duty Cycle/5, Delay/1
  Delay/1 -> Discrete-Time Integrator/2
  ADC Output 8 ADC samples on AN8 Synchronized with PWM (reducing conversion noise)/1 -> Sum of Elements Average/1
  Interrupt/1 -> Asynchronous Subsystem Update PWM channels to On / Off based on Hall sensor changes detected/Trigger
  Change Notification/1 -> Estimate Speed From CN period measured Protect for null speed/1(CN PER1)
  Rate Transition/1 -> Asynchronous Subsystem Update PWM channels to On / Off based on Hall sensor changes detected/1(Direction)
  Digital Input/1 -> Change when button is pressed/1
  Integer Delay3/1 -> Logical Operator/1
  Logical Operator/1 -> Integer Delay3/1, Rate Transition/1  "Toggle"
  Change when button is pressed/1 -> Logical Operator/2
  Ground/1 -> Update PWM duty Cycle/4
  Sum of Elements Average/1 -> Gain2/1  "U2 CH1"
  Sum1/1 -> Discrete-Time Integrator2/1, Gain1/1  "Speed Error (RPM)"
  Saturation/1 -> Update PWM duty Cycle/1, Update PWM duty Cycle/3, Update PWM duty Cycle/2, [command]  "cmd"
  Gain1/1 -> Sum2/1
  Discrete-Time Integrator2/1 -> Sum2/2
  Change Notification/3 -> Estimate Speed From CN period measured Protect for null speed/3(CN PER2)
  Change Notification/5 -> Estimate Speed From CN period measured Protect for null speed/5(CN PER3)
  Change Notification/6 -> Estimate Speed From CN period measured Protect for null speed/6(Rise Event 3)
  Change Notification/4 -> Estimate Speed From CN period measured Protect for null speed/4(Rise Event 2)
  Change Notification/2 -> Estimate Speed From CN period measured Protect for null speed/2(Rise Event 1)
  Estimate Speed From CN period measured Protect for null speed/1(Measured Speed) -> [SpeedFeedback], Sum1/2  "Feedback"
  Gain2/1 -> [SetPoint], Sum1/1  "Speed set point (RPM)"
  MCU Load Output mcu run time for 10 times steps/1 -> UART Tx-Matlab1/1  "U2 CH4"
  [SetPoint] -> UART Tx-Matlab/1  "U2 CH1"
  [SpeedFeedback] -> Data Type Conversion to RPM1/1  "U2 CH2"
  [command] -> UART Tx-Matlab/3  "U2 CH3"
  Delay1/1 -> Discrete-Time Integrator2/2
  Sum2/1 -> Saturation/1
  Data Type Conversion to RPM1/1 -> UART Tx-Matlab/2  "U2 CH2"

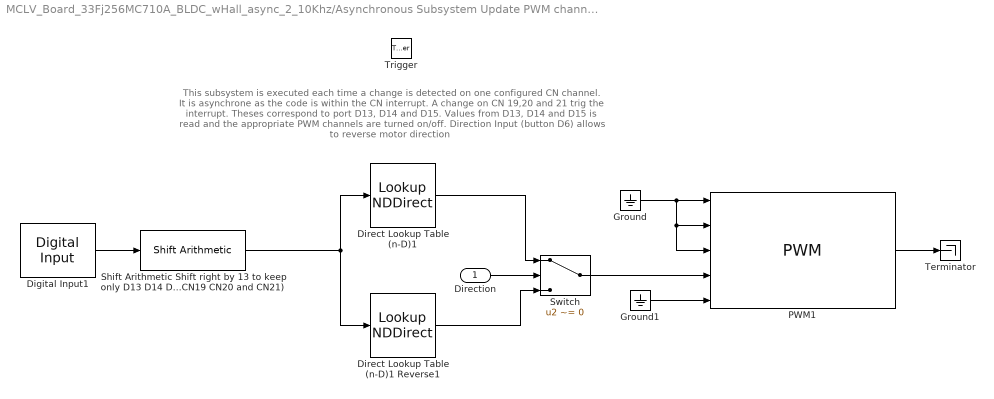
== system MCLV_Board_33Fj256MC710A_BLDC_wHall_async_2_10Khz/Asynchronous Subsystem Update PWM channels to On / Off based on Hall sensor changes detected ==
  note: This subsystem is executed each time a change is detected on one configured CN channel.
      | It is asynchrone as the code is within the CN interrupt.
      | A change on CN 19,20 and 21 trig the interrupt. Theses correspond to port D13, D14 and D15.
      | Values from D13, D14 and D15 is read and the appropriate PWM channels are turned on/off.
      |
      | Direction Input (button D6) allows to reverse motor direction
  Direction : Inport
  Trigger : TriggerPort  TriggerType=function-call  PortDimensions=1
  Digital Input1 : MCHP_Blockset/Digital IO/Digital Input  PORT=Dynamic Options  PORT_TXT="D   [ 0 : 15 ]"  PIN=[13 14 15]  PACK=on  SIMULTANEOUS=off  ORDERING=None  SampleTime=-1  MCHP_PORT={Digital In}{DIN}2:0:D13;{Digital In}{DIN}2:0:D14;{Digital In}{DIN}2:0:D15;  MCHP_MASTERLINK=MCLV_Board_33Fj256MC710A_BLDC_wHall_async_2_10Khz/Microchip Master
  Direct Lookup Table (n-D)1 : LookupNDDirect  NumberOfTableDimensions=1  Table=[0 8193 516 8196 2064 2049 528 0]  TableDataTypeStr=uint16
  Direct Lookup Table (n-D)1 Reverse1 : LookupNDDirect  NumberOfTableDimensions=1  Table=[0 528 2049 2064 8196 516 8193 0]  TableDataTypeStr=uint16
  Ground : Ground
  Ground1 : Ground
  PWM1 : MCHP_Blockset/PWM IO/PWM  PWM_REF=Duplicate ports for PWM 1  ChannelHighLowChk=off  Channel="[1  2 3]"  ChannelHigh=[1 2 4]  InitialPeriod=.001/8  InputPeriodeChk=off  CAM=off  IUE=off  Info="PWM1max = 9997  ;   % ==>  13.2873 bits"  MCHP_MASTERLINK=MCLV_Board_33Fj256MC710A_BLDC_wHall_async_2_10Khz/Microchip Master  SampleTime=-1  DeadTimePrescaleA=2e-6  DeadTimePrescaleB=0  DTPWM1a=Prescaler A  DTPWM1i=Prescaler A  DTPWM2a=Prescaler A  DTPWM2i=Prescaler A  DTPWM3a=Prescaler A  DTPWM3i=Prescaler A  DTPWM4a=Prescaler A  DTPWM4i=Prescaler A  PIN_FaultA=Dynamic Options  PIN_FaultA_TXT=<empty>  FAULTA_FLATM=Use Re-Enable block input after Fault is detected  FaultA_Output=on  FaultA_PWM1_State=H/L ==> 00  FaultA_PWM2_State=H/L ==> 00  FaultA_PWM3_State=H/L ==> 00  FaultA_PWM4_State=No Changes (PWM)  PIN_FaultB=Dynamic Options  PIN_FaultB_TXT=<empty>  FAULTB_FLBTM=Use Re-Enable block input after Fault is detected  FaultB_Output=off  FaultB_PWM1_State=No Changes (PWM)  FaultB_PWM2_State=No Changes (PWM)  FaultB_PWM3_State=No Changes (PWM)  FaultB_PWM4_State=No Changes (PWM)  PxSECMP=0  PxSECMPBlkInChk=off  OVDCONChk=on
  Shift Arithmetic Shift right by 13 to keep only D13 D14 D15 (CN19 CN20 and CN21) : simulink/Logic and Bit Operations/Shift Arithmetic  SystemSampleTime=-1  nBitShiftRight=13  nBinPtShiftRight=0
  Switch : Switch  Criteria=u2 ~= 0
  Terminator : Terminator
  wires:
  Ground/1 -> PWM1/1, PWM1/2, PWM1/3
  Ground1/1 -> PWM1/5
  PWM1/1 -> Terminator/1
  Shift Arithmetic Shift right by 13 to keep only D13 D14 D15 (CN19 CN20 and CN21)/1 -> Direct Lookup Table (n-D)1 Reverse1/1, Direct Lookup Table (n-D)1/1
  Direct Lookup Table (n-D)1 Reverse1/1 -> Switch/3
  Direct Lookup Table (n-D)1/1 -> Switch/1
  Direction/1 -> Switch/2
  Switch/1 -> PWM1/4
  Digital Input1/1 -> Shift Arithmetic Shift right by 13 to keep only D13 D14 D15 (CN19 CN20 and CN21)/1

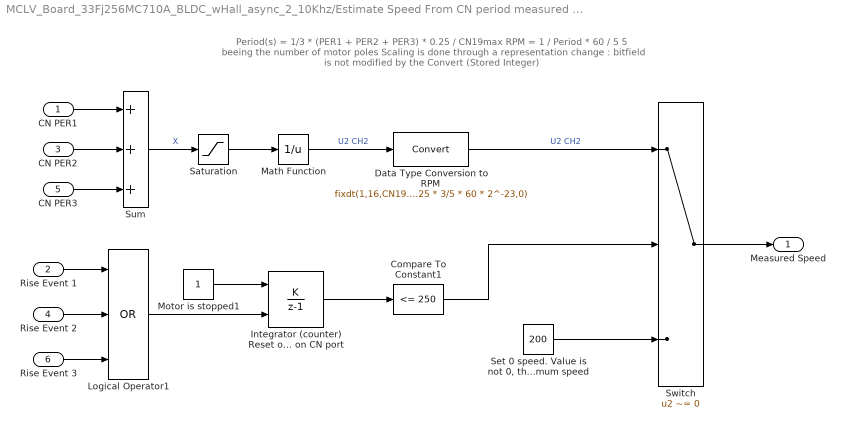
== system MCLV_Board_33Fj256MC710A_BLDC_wHall_async_2_10Khz/Estimate Speed From CN period measured Protect for null speed ==
  note: Period(s) = 1/3 * (PER1 + PER2 + PER3)  *  0.25 / CN19max
      | RPM = 1 / Period * 60 / 5
      | 5 beeing the number of motor poles
      | Scaling is done through a representation change :
      |   bitfield is not modified by the Convert (Stored Integer)
  CN PER1 : Inport
  Rise Event 1 : Inport  Port=2
  CN PER2 : Inport  Port=3
  Rise Event 2 : Inport  Port=4
  CN PER3 : Inport  Port=5
  Rise Event 3 : Inport  Port=6
  Compare To Constant1 : simulink/Logic and Bit Operations/Compare To Constant  SystemSampleTime=-1  relop=<=  const=250  LogicOutDataTypeMode=boolean
  Data Type Conversion to RPM : DataTypeConversion  OutDataTypeMode=Specify via dialog  OutDataType=fixdt(1,16,CN19max/0.25 * 3/5 * 60 * 2^-23,0)  OutDataTypeStr=fixdt(1,16,CN19max/0.25 * 3/5 * 60 * 2^-23,0)  ConvertRealWorld=Stored Integer (SI)
  Integrator (counter) Reset on each rise edge detected on CN port : DiscreteIntegrator  IntegratorMethod=Accumulation: Forward Euler  gainval=1  ExternalReset=level  SampleTime=-1  OutDataTypeMode=uint16  OutDataTypeStr=uint16  SaturateOnIntegerOverflow=on  LimitOutput=on  UpperSaturationLimit=255  LowerSaturationLimit=0  ICPrevOutput=DiscIntNeverNeededParam  ICPrevScaledInput=DiscIntNeverNeededParam
  Logical Operator1 : Logic  Operator=OR  Inputs=3  AllPortsSameDT=off  OutDataTypeMode=boolean  OutDataTypeStr=boolean
  Math Function : Math  Operator=reciprocal  OutputSignalType=real  OutDataTypeMode=Specify via dialog  OutDataType=fixdt(0,16,23)  OutDataTypeStr=fixdt(0,16,23)  SaturateOnIntegerOverflow=on
  Motor is stopped1 : Constant  OutDataTypeStr=Inherit: Inherit via back propagation
  Saturation : Saturate  UpperLimit=65535  LowerLimit=1  OutDataTypeMode=uint16  OutDataTypeStr=uint16
  "Set 0 speed. Value is not 0, thus If set point (from ADC) is lower than this low value, The controller will drive PWM to 0. This value set the minimum speed" : Constant  Value=200  OutDataTypeStr=Inherit: Inherit via back propagation
  Sum : Sum  Inputs=+++  RndMeth=Simplest  SaturateOnIntegerOverflow=on  OutDataTypeStr=Inherit: Same as first input
  Switch : Switch  Criteria=u2 ~= 0
  Measured Speed : Outport
  wires:
  Sum/1 -> Saturation/1  "X"
  Math Function/1 -> Data Type Conversion to RPM/1  "U2 CH2"
  Saturation/1 -> Math Function/1
  Logical Operator1/1 -> Integrator (counter) Reset on each rise edge detected on CN port/2
  Motor is stopped1/1 -> Integrator (counter) Reset on each rise edge detected on CN port/1
  Integrator (counter) Reset on each rise edge detected on CN port/1 -> Compare To Constant1/1
  Compare To Constant1/1 -> Switch/2
  Data Type Conversion to RPM/1 -> Switch/1  "U2 CH2"
  "Set 0 speed. Value is not 0, thus If set point (from ADC) is lower than this low value, The controller will drive PWM to 0. This value set the minimum speed"/1 -> Switch/3
  CN PER1/1 -> Sum/1
  CN PER2/1 -> Sum/2
  CN PER3/1 -> Sum/3
  Switch/1 -> Measured Speed/1
  Rise Event 1/1 -> Logical Operator1/1
  Rise Event 2/1 -> Logical Operator1/2
  Rise Event 3/1 -> Logical Operator1/3
